simulink model "H8_6GDL_nolineal"  (R2022b)
settings: Solver=FixedStepAuto  StartTime=0.0  StopTime=5  FixedStep=1/7500  MaxStep=1e-3  RelTol=1e-3
InitFcn:
  | load("ems.mat");
  | load("hems.mat");
  | load('fuerzasY_LIM.mat')
  | load('matrices_linealizacion_6gdl.mat')
  | m = 200;
  | g = 9.81;
  | 
  | x_lev12 = 0.50086;
  | x_lev34 = 0.48414;
  | x_guid12 = 0.50503;
  | x_guid34 = 0.48831;
  | x_lim = 0.00778;
  | 
  | y_lev13 = 0.23523;
  | y_lev24 = 0.23827;
  | y_guid13 = 0.2372;
  | y_guid24 = 0.2402;
  | y_lim = 0.00154;
  | y_brk = 0.21552;
  | 
  | z_lev = 0.07138;
  | z_guid = 0.04113;
  | z_lim = 0.09146;
  | z_brk = 0.03941;
  | 
  | kp_lev = 50;
  | ki_lev = 400;
  | kp_guid = 6;
  | ki_guid = 46.5;
  | 
  | Imax_lev = 50;
  | Imin_lev = -50;
  | Imax_guid = 50;
  | Imin_guid = 0;
  | 
  | cg_nom=0.61448;
  | lev_nom=0.01965;
  | cg_suelo=0.61733;
  | cg_techo=0.60483;
  | 
  | I = [43.082 0 0; 0 26.887 -0; 0 0 29.297];
  | 
  | fs_current = 20000;
  | fl_current = 10000;
  | var_current = 0.052125100064495;
  | offset_current = 0.001065378087271;
  | 
  | fs_airgap = 20000;
  | fl_airgap = 7500;
  | var_airgap = 1.112140361208638e-08;
  | offset_airgap = 0;
  | airgap_min = 80/1000;
  | airgap_max = 115/1000;
  | 
  | current_filter_order = 20;
  | 
  | airgap_filter_order = 20;
  | N=16;
values from neighbouring files (symbols this model uses):
  A6 = [0 0 0 0 0 0 0 0 0 0 0 0 ... (100 elements, 10x10)]    [matrices_linealizacion_6gdl.mat]    (also in matrices_linealizacion_6gdl2.mat)
  B6 = [0 0 0 0 0 0 -0.0459993641186 -0.0505798680894 0.151580453785 0 0 0 ... (80 elements, 10x8)]    [matrices_linealizacion_6gdl.mat]    (also in matrices_linealizacion_6gdl2.mat)
  C6 = [1 0 0 0 0 0 0 0 0 0 0 1 ... (100 elements, 10x10)]    [matrices_linealizacion_6gdl.mat]    (also in matrices_linealizacion_6gdl2.mat)
  current = [0 10 20 30 40 50 60 70 80 90 100]    [fuerzasY_LIM.mat]
  D6 = [0 0 0 0 0 0 0 0 0 0 0 0 ... (80 elements, 10x8)]    [matrices_linealizacion_6gdl.mat]    (also in matrices_linealizacion_6gdl2.mat)
  FuerzaRail_Y = [0 0 0 0 0 0 0 0.015951701 0.168531476 0.364402347 0.577209778 0.832001165 ... (77 elements, 7x11)]    [fuerzasY_LIM.mat]
  hems =     [hems.mat]
  Ka = [0 0 0 0 4539.83149439 -4539.83149439 4539.83149439 -4539.83149439 -5130.48383819 -5130.48383819 -5130.48383819 -5130.48383819 ... (120 elements, 8x15)]    [Ka_reajustada.mat]    (also in matrices_linealizacion_6gdl.mat = [0 0 0 0 6002.75566687 -6002.75566687 6002.75566687 -6002.75; matrices_linealizacion_6gdl2.mat = [0 0 0 0 1200.55113337 -1200.55113337 1200.55113337 -1200.55)
  Y = [0 1 2 3 4 5 6]    [fuerzasY_LIM.mat]
undefined symbols (not defined in the file or in its folder): DiscIntNeverNeededParam, ems, magnitude
libraries: slpidlib x16, simulink x5
(part 2 of 2)

== system H8_6GDL_nolineal/EMS/RL ==
  target voltage : Inport
  airgap : Inport  Port=2
  temperature : Inport  Port=3
  2-D Lookup Table : Lookup_n-D  BreakpointsForDimension1=ems.Airgap  BreakpointsForDimension2=ems.Flux_Current(2:55)  Table=ems.Inductance  InternalRulePriority=Speed  RndMeth=Simplest
      settings: InputPortMap=u0,u1
  Abs : Abs  SaturateOnIntegerOverflow=off
  Add : Sum  Inputs=+-
  Delay{,1..3} (4 alike) : Delay  DelayLength=1
  Divide : Product  Inputs=*/
  Divide1 : Product  Inputs=*/
  Divide2 : Product  Inputs=*/
  Integrator1 : Integrator
  Subsystem : Subsystem
  to mm : Gain  Gain=1000
  current : Outport
  wires:
  airgap/1 -> to mm/1
  Divide/1 -> Integrator1/1
  Add/1 -> Divide/1
  Integrator1/1 -> Abs/1, current/1, Delay3/1, Add/2  "current applied"
  2-D Lookup Table/1 -> Divide2/1  "L"
  target voltage/1 -> Divide1/1
  temperature/1 -> Delay2/1
  Divide1/1 -> Add/1
  Subsystem/1(R) -> Divide2/2, Divide1/2  "R"
  Delay3/1 -> Subsystem/1(Current)
  Delay2/1 -> Subsystem/2(Temperature)
  Divide2/1 -> Divide/2
  Delay1/1 -> 2-D Lookup Table/2
  Delay/1 -> 2-D Lookup Table/1
  Abs/1 -> Delay1/1
  to mm/1 -> Delay/1

== system H8_6GDL_nolineal/EMS/RL1 ==
  target voltage : Inport
  airgap : Inport  Port=2
  temperature : Inport  Port=3
  2-D Lookup Table : Lookup_n-D  BreakpointsForDimension1=ems.Airgap  BreakpointsForDimension2=ems.Flux_Current(2:55)  Table=ems.Inductance  InternalRulePriority=Speed  RndMeth=Simplest
      settings: InputPortMap=u0,u1
  Abs : Abs  SaturateOnIntegerOverflow=off
  Add : Sum  Inputs=+-
  Delay{,1..3} (4 alike) : Delay  DelayLength=1
  Divide : Product  Inputs=*/
  Divide1 : Product  Inputs=*/
  Divide2 : Product  Inputs=*/
  Integrator1 : Integrator
  Subsystem : Subsystem
  to mm : Gain  Gain=1000
  current : Outport
  wires:
  airgap/1 -> to mm/1
  Divide/1 -> Integrator1/1
  Add/1 -> Divide/1
  Integrator1/1 -> Abs/1, current/1, Delay3/1, Add/2  "current applied"
  2-D Lookup Table/1 -> Divide2/1  "L"
  target voltage/1 -> Divide1/1
  temperature/1 -> Delay2/1
  Divide1/1 -> Add/1
  Subsystem/1(R) -> Divide2/2, Divide1/2  "R"
  Delay3/1 -> Subsystem/1(Current)
  Delay2/1 -> Subsystem/2(Temperature)
  Divide2/1 -> Divide/2
  Delay1/1 -> 2-D Lookup Table/2
  Delay/1 -> 2-D Lookup Table/1
  Abs/1 -> Delay1/1
  to mm/1 -> Delay/1

== system H8_6GDL_nolineal/EMS/RL2 ==
  target voltage : Inport
  airgap : Inport  Port=2
  temperature : Inport  Port=3
  2-D Lookup Table : Lookup_n-D  BreakpointsForDimension1=ems.Airgap  BreakpointsForDimension2=ems.Flux_Current(2:55)  Table=ems.Inductance  InternalRulePriority=Speed  RndMeth=Simplest
      settings: InputPortMap=u0,u1
  Abs : Abs  SaturateOnIntegerOverflow=off
  Add : Sum  Inputs=+-
  Delay{,1..3} (4 alike) : Delay  DelayLength=1
  Divide : Product  Inputs=*/
  Divide1 : Product  Inputs=*/
  Divide2 : Product  Inputs=*/
  Integrator1 : Integrator
  Subsystem : Subsystem
  to mm : Gain  Gain=1000
  current : Outport
  wires:
  airgap/1 -> to mm/1
  Divide/1 -> Integrator1/1
  Add/1 -> Divide/1
  Integrator1/1 -> Abs/1, current/1, Delay3/1, Add/2  "current applied"
  2-D Lookup Table/1 -> Divide2/1  "L"
  target voltage/1 -> Divide1/1
  temperature/1 -> Delay2/1
  Divide1/1 -> Add/1
  Subsystem/1(R) -> Divide2/2, Divide1/2  "R"
  Delay3/1 -> Subsystem/1(Current)
  Delay2/1 -> Subsystem/2(Temperature)
  Divide2/1 -> Divide/2
  Delay1/1 -> 2-D Lookup Table/2
  Delay/1 -> 2-D Lookup Table/1
  Abs/1 -> Delay1/1
  to mm/1 -> Delay/1

== system H8_6GDL_nolineal/EMS/RL3 ==
  target voltage : Inport
  airgap : Inport  Port=2
  temperature : Inport  Port=3
  2-D Lookup Table : Lookup_n-D  BreakpointsForDimension1=ems.Airgap  BreakpointsForDimension2=ems.Flux_Current(2:55)  Table=ems.Inductance  InternalRulePriority=Speed  RndMeth=Simplest
      settings: InputPortMap=u0,u1
  Abs : Abs  SaturateOnIntegerOverflow=off
  Add : Sum  Inputs=+-
  Delay{,1..3} (4 alike) : Delay  DelayLength=1
  Divide : Product  Inputs=*/
  Divide1 : Product  Inputs=*/
  Divide2 : Product  Inputs=*/
  Integrator1 : Integrator
  Subsystem : Subsystem
  to mm : Gain  Gain=1000
  current : Outport
  wires:
  airgap/1 -> to mm/1
  Divide/1 -> Integrator1/1
  Add/1 -> Divide/1
  Integrator1/1 -> Abs/1, current/1, Delay3/1, Add/2  "current applied"
  2-D Lookup Table/1 -> Divide2/1  "L"
  target voltage/1 -> Divide1/1
  temperature/1 -> Delay2/1
  Divide1/1 -> Add/1
  Subsystem/1(R) -> Divide2/2, Divide1/2  "R"
  Delay3/1 -> Subsystem/1(Current)
  Delay2/1 -> Subsystem/2(Temperature)
  Divide2/1 -> Divide/2
  Delay1/1 -> 2-D Lookup Table/2
  Delay/1 -> 2-D Lookup Table/1
  Abs/1 -> Delay1/1
  to mm/1 -> Delay/1

== system H8_6GDL_nolineal/EMS/Subsystem1 ==
  current5 : Inport
  Constant : Constant  Value=0
  Constant2 : Constant  Value=50
  Switch : Switch  Criteria=u2 > Threshold  SaturateOnIntegerOverflow=off  InputSameDT=off
  Switch1 : Switch  Criteria=u2 > Threshold  Threshold=50  SaturateOnIntegerOverflow=off  InputSameDT=off
  Out1 : Outport
  wires:
  current5/1 -> Switch/1, Switch/2
  Switch1/1 -> Out1/1
  Switch/1 -> Switch1/3, Switch1/2
  Constant/1 -> Switch/3
  Constant2/1 -> Switch1/1

== system H8_6GDL_nolineal/HEMS1/RL ==
  target voltage : Inport
  airgap : Inport  Port=2
  temperature : Inport  Port=3
  2-D Lookup Table : Lookup_n-D  BreakpointsForDimension1=hems.Airgap  BreakpointsForDimension2=hems.Current(2:110)  Table=hems.Inductance  InternalRulePriority=Speed  RndMeth=Simplest
      settings: InputPortMap=u0,u1
  Add : Sum  Inputs=+-
  Delay{1..4} (4 alike) : Delay  DelayLength=1
  Divide : Product  Inputs=*/
  Divide1 : Product  Inputs=*/
  Divide2 : Product  Inputs=*/
  Integrator1 : Integrator
  Rate Transition : RateTransition  Commented=through
  Saturation5 : Saturate  UpperLimit=0.0225  LowerLimit=0.01
  Subsystem : Subsystem
  to mm : Gain  Gain=1000
  current : Outport
  wires:
  airgap/1 -> Saturation5/1
  Divide/1 -> Integrator1/1
  Add/1 -> Divide/1
  Integrator1/1 -> Delay1/1, current/1, Delay3/1, Add/2  "current applied"
  2-D Lookup Table/1 -> Divide2/1  "L"
  temperature/1 -> Delay2/1
  Divide1/1 -> Add/1
  Subsystem/1(R) -> Divide2/2, Divide1/2  "R"
  Delay3/1 -> Subsystem/1(Current)
  Delay2/1 -> Subsystem/2(Temperature)
  Divide2/1 -> Divide/2
  Delay1/1 -> 2-D Lookup Table/2
  Rate Transition/1 -> 2-D Lookup Table/1
  Saturation5/1 -> to mm/1
  to mm/1 -> Delay4/1
  Delay4/1 -> Rate Transition/1
  target voltage/1 -> Divide1/1

== system H8_6GDL_nolineal/HEMS1/RL1 ==
  target current : Inport
  airgap : Inport  Port=2
  temperature : Inport  Port=3
  2-D Lookup Table : Lookup_n-D  BreakpointsForDimension1=hems.Airgap  BreakpointsForDimension2=hems.Current(2:110)  Table=hems.Inductance  InternalRulePriority=Speed  RndMeth=Simplest
      settings: InputPortMap=u0,u1
  Add : Sum  Inputs=+-
  Delay{1..4} (4 alike) : Delay  DelayLength=1
  Divide : Product  Inputs=*/
  Divide1 : Product  Inputs=*/
  Divide2 : Product  Inputs=*/
  Integrator1 : Integrator
  Rate Transition : RateTransition  Commented=through
  Saturation1 : Saturate  UpperLimit=0.0225  LowerLimit=0.01
  Subsystem : Subsystem
  to mm : Gain  Gain=1000
  current : Outport
  wires:
  airgap/1 -> Saturation1/1
  Divide/1 -> Integrator1/1
  Add/1 -> Divide/1
  Integrator1/1 -> Delay1/1, current/1, Delay3/1, Add/2  "current applied"
  2-D Lookup Table/1 -> Divide2/1  "L"
  target current/1 -> Divide1/1
  temperature/1 -> Delay2/1
  Divide1/1 -> Add/1
  Subsystem/1(R) -> Divide2/2, Divide1/2  "R"
  Delay3/1 -> Subsystem/1(Current)
  Delay2/1 -> Subsystem/2(Temperature)
  Divide2/1 -> Divide/2
  Delay1/1 -> 2-D Lookup Table/2
  Rate Transition/1 -> 2-D Lookup Table/1
  Saturation1/1 -> to mm/1
  to mm/1 -> Delay4/1
  Delay4/1 -> Rate Transition/1

== system H8_6GDL_nolineal/HEMS1/RL2 ==
  target current : Inport
  airgap : Inport  Port=2
  temperature : Inport  Port=3
  2-D Lookup Table : Lookup_n-D  BreakpointsForDimension1=hems.Airgap  BreakpointsForDimension2=hems.Current(2:110)  Table=hems.Inductance  InternalRulePriority=Speed  RndMeth=Simplest
      settings: InputPortMap=u0,u1
  Add : Sum  Inputs=+-
  Delay{1..4} (4 alike) : Delay  DelayLength=1
  Divide : Product  Inputs=*/
  Divide1 : Product  Inputs=*/
  Divide2 : Product  Inputs=*/
  Integrator1 : Integrator
  Rate Transition : RateTransition  Commented=through
  Saturation5 : Saturate  UpperLimit=0.0225  LowerLimit=0.01
  Subsystem : Subsystem
  to mm : Gain  Gain=1000
  current : Outport
  wires:
  airgap/1 -> Saturation5/1
  Divide/1 -> Integrator1/1
  Add/1 -> Divide/1
  Integrator1/1 -> Delay1/1, current/1, Delay3/1, Add/2  "current applied"
  2-D Lookup Table/1 -> Divide2/1  "L"
  target current/1 -> Divide1/1
  temperature/1 -> Delay2/1
  Divide1/1 -> Add/1
  Subsystem/1(R) -> Divide2/2, Divide1/2  "R"
  Delay3/1 -> Subsystem/1(Current)
  Delay2/1 -> Subsystem/2(Temperature)
  Divide2/1 -> Divide/2
  Delay1/1 -> 2-D Lookup Table/2
  Rate Transition/1 -> 2-D Lookup Table/1
  Saturation5/1 -> to mm/1
  to mm/1 -> Delay4/1
  Delay4/1 -> Rate Transition/1

== system H8_6GDL_nolineal/HEMS1/RL3 ==
  target current : Inport
  airgap : Inport  Port=2
  temperature : Inport  Port=3
  2-D Lookup Table : Lookup_n-D  BreakpointsForDimension1=hems.Airgap  BreakpointsForDimension2=hems.Current(2:110)  Table=hems.Inductance  InternalRulePriority=Speed  RndMeth=Simplest
      settings: InputPortMap=u0,u1
  Add : Sum  Inputs=+-
  Delay{1..4} (4 alike) : Delay  DelayLength=1
  Divide : Product  Inputs=*/
  Divide1 : Product  Inputs=*/
  Divide2 : Product  Inputs=*/
  Integrator1 : Integrator
  Rate Transition : RateTransition  Commented=through
  Saturation5 : Saturate  UpperLimit=0.0225  LowerLimit=0.01
  Subsystem : Subsystem
  to mm : Gain  Gain=1000
  current : Outport
  wires:
  airgap/1 -> Saturation5/1
  Divide/1 -> Integrator1/1
  Add/1 -> Divide/1
  Integrator1/1 -> Delay1/1, current/1, Delay3/1, Add/2  "current applied"
  2-D Lookup Table/1 -> Divide2/1  "L"
  target current/1 -> Divide1/1
  temperature/1 -> Delay2/1
  Divide1/1 -> Add/1
  Subsystem/1(R) -> Divide2/2, Divide1/2  "R"
  Delay3/1 -> Subsystem/1(Current)
  Delay2/1 -> Subsystem/2(Temperature)
  Divide2/1 -> Divide/2
  Delay1/1 -> 2-D Lookup Table/2
  Rate Transition/1 -> 2-D Lookup Table/1
  Saturation5/1 -> to mm/1
  to mm/1 -> Delay4/1
  Delay4/1 -> Rate Transition/1

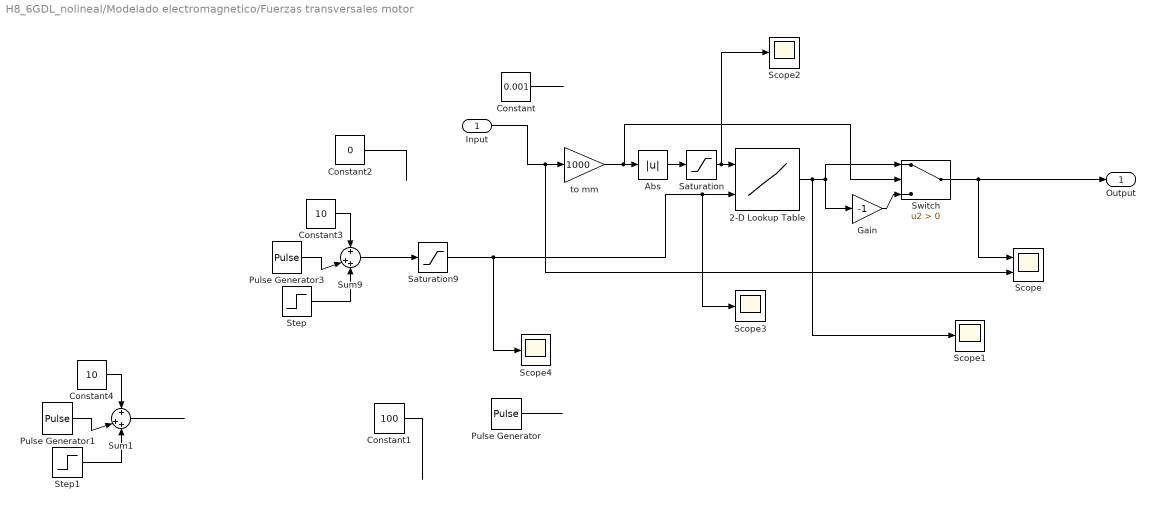
== system H8_6GDL_nolineal/Modelado electromagnetico/Fuerzas transversales motor ==
  Input : Inport
  2-D Lookup Table : Lookup_n-D  BreakpointsForDimension1=Y  BreakpointsForDimension2=current  Table=FuerzaRail_Y  InternalRulePriority=Speed  RndMeth=Simplest
      settings: InputPortMap=u0,u1
  Abs : Abs  SaturateOnIntegerOverflow=off
  Constant : Constant  Value=0.001
  Constant1 : Constant  Value=100
  Constant2 : Constant  Value=0
  Constant3 : Constant  Value=10
  Constant4 : Constant  Value=10
  Gain : Gain  Gain=-1
  Pulse Generator : DiscretePulseGenerator  PulseType=Time based  Amplitude=100  PulseWidth=75  PhaseDelay=3
  Pulse Generator1 : DiscretePulseGenerator  PulseType=Time based  Amplitude=100  PulseWidth=95  PhaseDelay=4.2
  Pulse Generator3 : DiscretePulseGenerator  PulseType=Time based  Amplitude=100  PulseWidth=95  PhaseDelay=1
  Saturation : Saturate  UpperLimit=6  LowerLimit=0
  Saturation9 : Saturate  UpperLimit=100  LowerLimit=0
  Scope : Scope  NumInputPorts=2
  Scope{1..4} (4 alike) : Scope
  Step : Step  Time=5  After=-100  SampleTime=0
  Step1 : Step  Time=8.2  After=-100  SampleTime=0
  Sum1 : Sum  Inputs=+|++
  Sum9 : Sum  Inputs=+|++
  Switch : Switch  Criteria=u2 > Threshold  SaturateOnIntegerOverflow=off  InputSameDT=off
  to mm : Gain  Gain=1000
  Output : Outport
  wires:
  Constant/1 -> ?
  Input/1 -> to mm/1, Scope/2
  Gain/1 -> Switch/3
  Abs/1 -> Saturation/1
  to mm/1 -> Switch/2, Abs/1
  2-D Lookup Table/1 -> Scope1/1, Gain/1, Switch/1
  Saturation9/1 -> Scope4/1, Scope3/1, 2-D Lookup Table/2
  Switch/1 -> Output/1, Scope/1
  Saturation/1 -> Scope2/1, 2-D Lookup Table/1
  Pulse Generator/1 -> ?
  Constant1/1 -> ?
  Constant2/1 -> ?
  Sum9/1 -> Saturation9/1
  Pulse Generator3/1 -> Sum9/2
  Constant3/1 -> Sum9/1
  Step/1 -> Sum9/3
  Constant4/1 -> Sum1/1
  Step1/1 -> Sum1/3
  Pulse Generator1/1 -> Sum1/2
  Sum1/1 -> ?

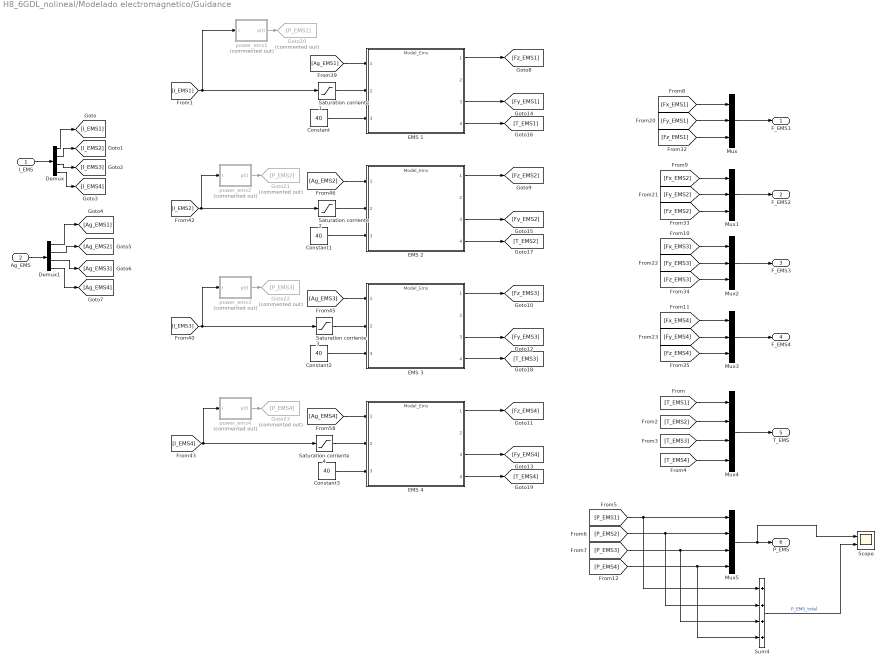
== system H8_6GDL_nolineal/Modelado electromagnetico/Guidance ==
  I_EMS : Inport
  Ag_EMS : Inport  Port=2
  Constant{,1..3} (4 alike) : Constant  Value=40
  Demux : Demux
  Demux1 : Demux
  EMS {1..4} (4 alike) : ModelReference  ModelNameDialog=Model_Ems.slx  SimulationMode=Normal  ModelReferenceVersion=1.24
  Goto20 : Goto  Commented=on  GotoTag=P_EMS1
  Goto21 : Goto  Commented=on  GotoTag=P_EMS2
  Goto22 : Goto  Commented=on  GotoTag=P_EMS3
  Goto23 : Goto  Commented=on  GotoTag=P_EMS4
  Mux{,1..3} (4 alike) : Mux  Inputs=3
  Mux4 : Mux
  Mux5 : Mux
  Saturation corriente {1..4} (4 alike) : Saturate  UpperLimit=Imax_guid  LowerLimit=Imin_guid
  Scope : Scope  NumInputPorts=2
  Sum4 : Sum  Inputs=++++
  power_ems1 : Subsystem  Commented=on
  power_ems2 : Subsystem  Commented=on
  power_ems3 : Subsystem  Commented=on
  power_ems4 : Subsystem  Commented=on
  F_EMS1 : Outport
  F_EMS2 : Outport  Port=2
  F_EMS3 : Outport  Port=3
  F_EMS4 : Outport  Port=4
  T_EMS : Outport  Port=5
  P_EMS : Outport  Port=6
  wires:
  [Fz_EMS4] -> Mux3/3
  Demux1/4 -> [Ag_EMS4]
  [Fy_EMS1] -> Mux/2
  I_EMS/1 -> Demux/1
  Mux1/1 -> F_EMS2/1
  Demux/2 -> [I_EMS2]
  [Fy_EMS3] -> Mux2/2
  Mux3/1 -> F_EMS4/1
  [Fy_EMS4] -> Mux3/2
  [Fz_EMS1] -> Mux/3
  Mux/1 -> F_EMS1/1
  Mux2/1 -> F_EMS3/1
  [Fx_EMS3] -> Mux2/1
  Demux1/3 -> [Ag_EMS3]
  Ag_EMS/1 -> Demux1/1
  [Fz_EMS3] -> Mux2/3
  Demux/1 -> [I_EMS1]
  [Fz_EMS2] -> Mux1/3
  [Fx_EMS1] -> Mux/1
  Demux1/1 -> [Ag_EMS1]
  Demux/4 -> [I_EMS4]
  [Fx_EMS2] -> Mux1/1
  [Fy_EMS2] -> Mux1/2
  [Fx_EMS4] -> Mux3/1
  Demux/3 -> [I_EMS3]
  Demux1/2 -> [Ag_EMS2]
  EMS 1/3 -> [Fy_EMS1]
  [Ag_EMS4] -> EMS 4/1
  EMS 4/3 -> [Fy_EMS4]
  EMS 4/1 -> [Fz_EMS4]
  EMS 2/1 -> [Fz_EMS2]
  EMS 3/1 -> [Fz_EMS3]
  [Ag_EMS3] -> EMS 3/1
  Constant1/1 -> EMS 2/3
  Constant3/1 -> EMS 4/3
  Constant2/1 -> EMS 3/3
  Constant/1 -> EMS 1/3
  EMS 1/1 -> [Fz_EMS1]
  [Ag_EMS2] -> EMS 2/1
  EMS 3/3 -> [Fy_EMS3]
  EMS 2/3 -> [Fy_EMS2]
  [Ag_EMS1] -> EMS 1/1
  Mux4/1 -> T_EMS/1
  EMS 1/4 -> [T_EMS1]
  EMS 2/4 -> [T_EMS2]
  EMS 3/4 -> [T_EMS3]
  EMS 4/4 -> [T_EMS4]
  [T_EMS1] -> Mux4/1
  [T_EMS2] -> Mux4/2
  [T_EMS3] -> Mux4/3
  [T_EMS4] -> Mux4/4
  Saturation corriente 1/1 -> EMS 1/2
  Saturation corriente 2/1 -> EMS 2/2
  Saturation corriente 3/1 -> EMS 3/2
  Saturation corriente 4/1 -> EMS 4/2
  power_ems1/1(p(t)) -> Goto20/1
  power_ems2/1(p(t)) -> Goto21/1
  power_ems3/1(p(t)) -> Goto22/1
  power_ems4/1(p(t)) -> Goto23/1
  [P_EMS4] -> Sum4/4, Mux5/4
  [P_EMS1] -> Mux5/1, Sum4/1
  Sum4/1 -> Scope/2  "P_EMS_total"
  [P_EMS2] -> Mux5/2, Sum4/2
  Mux5/1 -> Scope/1, P_EMS/1
  [P_EMS3] -> Sum4/3, Mux5/3
  [I_EMS4] -> Saturation corriente 4/1, power_ems4/1(I)
  [I_EMS3] -> Saturation corriente 3/1, power_ems3/1(I)
  [I_EMS2] -> Saturation corriente 2/1, power_ems2/1(I)
  [I_EMS1] -> Saturation corriente 1/1, power_ems1/1(I)

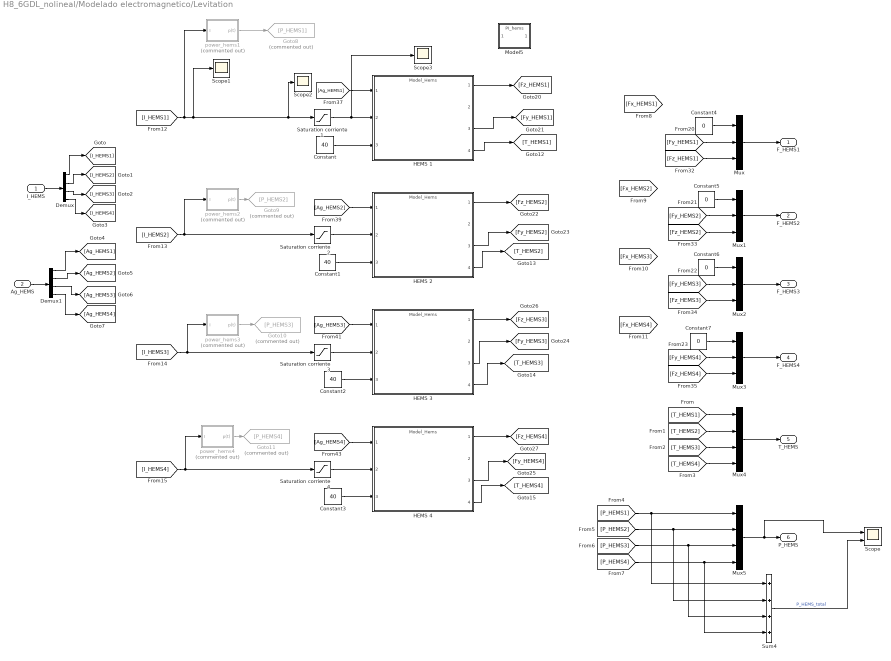
== system H8_6GDL_nolineal/Modelado electromagnetico/Levitation ==
  I_HEMS : Inport
  Ag_HEMS : Inport  Port=2
  Constant{,1..3} (4 alike) : Constant  Value=40
  Constant{4..7} (4 alike) : Constant  Value=0
  Demux : Demux
  Demux1 : Demux
  Goto10 : Goto  Commented=on  GotoTag=P_HEMS3
  Goto11 : Goto  Commented=on  GotoTag=P_HEMS4
  Goto8 : Goto  Commented=on  GotoTag=P_HEMS1
  Goto9 : Goto  Commented=on  GotoTag=P_HEMS2
  HEMS {1..4} (4 alike) : ModelReference  ModelNameDialog=Model_Hems.slx  SimulationMode=Normal  ModelReferenceVersion=1.27
  Model5 : ModelReference  ModelNameDialog=PI_hems.slx  SimulationMode=Normal  ModelReferenceVersion=1.6
  Mux{,1..3} (4 alike) : Mux  Inputs=3
  Mux4 : Mux
  Mux5 : Mux
  Saturation corriente {1..4} (4 alike) : Saturate  UpperLimit=Imax_lev  LowerLimit=Imin_lev
  Scope : Scope  NumInputPorts=2
  Scope1 : Scope
  Scope2 : Scope
  Scope3 : Scope
  Sum4 : Sum  Inputs=++++
  power_hems1 : Subsystem  Commented=on
  power_hems2 : Subsystem  Commented=on
  power_hems3 : Subsystem  Commented=on
  power_hems4 : Subsystem  Commented=on
  F_HEMS1 : Outport
  F_HEMS2 : Outport  Port=2
  F_HEMS3 : Outport  Port=3
  F_HEMS4 : Outport  Port=4
  T_HEMS : Outport  Port=5
  P_HEMS : Outport  Port=6
  wires:
  I_HEMS/1 -> Demux/1
  Mux/1 -> F_HEMS1/1
  Mux1/1 -> F_HEMS2/1
  Mux2/1 -> F_HEMS3/1
  Mux3/1 -> F_HEMS4/1
  Demux/1 -> [I_HEMS1]
  Demux/2 -> [I_HEMS2]
  Demux/3 -> [I_HEMS3]
  Demux/4 -> [I_HEMS4]
  Demux1/2 -> [Ag_HEMS2]
  Demux1/3 -> [Ag_HEMS3]
  Ag_HEMS/1 -> Demux1/1
  Demux1/4 -> [Ag_HEMS4]
  Demux1/1 -> [Ag_HEMS1]
  Constant4/1 -> Mux/1
  Constant5/1 -> Mux1/1
  Constant6/1 -> Mux2/1
  Constant7/1 -> Mux3/1
  [Fy_HEMS1] -> Mux/2
  [Fy_HEMS2] -> Mux1/2
  [Fy_HEMS3] -> Mux2/2
  [Fy_HEMS4] -> Mux3/2
  [Fz_HEMS1] -> Mux/3
  [Fz_HEMS2] -> Mux1/3
  [Fz_HEMS3] -> Mux2/3
  [Fz_HEMS4] -> Mux3/3
  [Ag_HEMS1] -> HEMS 1/1
  HEMS 1/1 -> [Fz_HEMS1]
  HEMS 1/3 -> [Fy_HEMS1]
  HEMS 2/3 -> [Fy_HEMS2]
  HEMS 2/1 -> [Fz_HEMS2]
  [Ag_HEMS2] -> HEMS 2/1
  HEMS 3/3 -> [Fy_HEMS3]
  HEMS 3/1 -> [Fz_HEMS3]
  [Ag_HEMS3] -> HEMS 3/1
  HEMS 4/3 -> [Fy_HEMS4]
  HEMS 4/1 -> [Fz_HEMS4]
  [Ag_HEMS4] -> HEMS 4/1
  Constant1/1 -> HEMS 2/3
  Constant2/1 -> HEMS 3/3
  Constant3/1 -> HEMS 4/3
  HEMS 1/4 -> [T_HEMS1]
  Constant/1 -> HEMS 1/3
  HEMS 2/4 -> [T_HEMS2]
  HEMS 3/4 -> [T_HEMS3]
  HEMS 4/4 -> [T_HEMS4]
  Mux4/1 -> T_HEMS/1
  [T_HEMS1] -> Mux4/1
  [T_HEMS4] -> Mux4/4
  [T_HEMS3] -> Mux4/3
  [T_HEMS2] -> Mux4/2
  Saturation corriente 1/1 -> Scope3/1, HEMS 1/2
  Saturation corriente 2/1 -> HEMS 2/2
  Saturation corriente 3/1 -> HEMS 3/2
  Saturation corriente 4/1 -> HEMS 4/2
  power_hems1/1(p(t)) -> Goto8/1
  [P_HEMS4] -> Sum4/4, Mux5/4
  [P_HEMS2] -> Mux5/2, Sum4/2
  [P_HEMS3] -> Sum4/3, Mux5/3
  Mux5/1 -> Scope/1, P_HEMS/1
  [P_HEMS1] -> Mux5/1, Sum4/1
  Sum4/1 -> Scope/2  "P_HEMS_total"
  power_hems2/1(p(t)) -> Goto9/1
  power_hems3/1(p(t)) -> Goto10/1
  power_hems4/1(p(t)) -> Goto11/1
  [I_HEMS4] -> Saturation corriente 4/1, power_hems4/1(I)
  [I_HEMS2] -> Saturation corriente 2/1, power_hems2/1(I)
  [I_HEMS1] -> power_hems1/1(I), Scope2/1, Saturation corriente 1/1, Scope1/1
  [I_HEMS3] -> Saturation corriente 3/1, power_hems3/1(I)

== system H8_6GDL_nolineal/Subsystem/Discr_Ampl ==
  señal : Inport
  Constant : Constant  Value=N
  Constant1 : Constant  Value=Max
  Constant2 : Constant  Value=Min
  MATLAB Function1 : MATLAB Function  TreatAsAtomicUnit=on
  señal_discretizada : Outport
  wires:
  MATLAB Function1/1(senal_discretizada) -> señal_discretizada/1
  señal/1 -> MATLAB Function1/1(senal)
  Constant1/1 -> MATLAB Function1/3(Max)
  Constant/1 -> MATLAB Function1/2(N)
  Constant2/1 -> MATLAB Function1/4(Min)

== system H8_6GDL_nolineal/Subsystem/Discr_Ampl1 ==
  señal : Inport
  Constant : Constant  Value=N
  Constant1 : Constant  Value=Max
  Constant2 : Constant  Value=Min
  MATLAB Function1 : MATLAB Function  TreatAsAtomicUnit=on
  señal_discretizada : Outport
  wires:
  MATLAB Function1/1(senal_discretizada) -> señal_discretizada/1
  señal/1 -> MATLAB Function1/1(senal)
  Constant1/1 -> MATLAB Function1/3(Max)
  Constant/1 -> MATLAB Function1/2(N)
  Constant2/1 -> MATLAB Function1/4(Min)

== system H8_6GDL_nolineal/Subsystem/Discr_Ampl2 ==
  señal : Inport
  Constant : Constant  Value=N
  Constant1 : Constant  Value=Max
  Constant2 : Constant  Value=Min
  MATLAB Function1 : MATLAB Function  TreatAsAtomicUnit=on
  señal_discretizada : Outport
  wires:
  MATLAB Function1/1(senal_discretizada) -> señal_discretizada/1
  señal/1 -> MATLAB Function1/1(senal)
  Constant1/1 -> MATLAB Function1/3(Max)
  Constant/1 -> MATLAB Function1/2(N)
  Constant2/1 -> MATLAB Function1/4(Min)

== system H8_6GDL_nolineal/Subsystem/Discr_Ampl3 ==
  señal : Inport
  Constant : Constant  Value=N
  Constant1 : Constant  Value=Max
  Constant2 : Constant  Value=Min
  MATLAB Function1 : MATLAB Function  TreatAsAtomicUnit=on
  señal_discretizada : Outport
  wires:
  MATLAB Function1/1(senal_discretizada) -> señal_discretizada/1
  señal/1 -> MATLAB Function1/1(senal)
  Constant1/1 -> MATLAB Function1/3(Max)
  Constant/1 -> MATLAB Function1/2(N)
  Constant2/1 -> MATLAB Function1/4(Min)

== system H8_6GDL_nolineal/Subsystem/Discr_Ampl4 ==
  señal : Inport
  Constant : Constant  Value=N
  Constant1 : Constant  Value=Max
  Constant2 : Constant  Value=Min
  MATLAB Function1 : MATLAB Function  TreatAsAtomicUnit=on
  señal_discretizada : Outport
  wires:
  MATLAB Function1/1(senal_discretizada) -> señal_discretizada/1
  señal/1 -> MATLAB Function1/1(senal)
  Constant1/1 -> MATLAB Function1/3(Max)
  Constant/1 -> MATLAB Function1/2(N)
  Constant2/1 -> MATLAB Function1/4(Min)

== system H8_6GDL_nolineal/Subsystem/Discr_Ampl5 ==
  señal : Inport
  Constant : Constant  Value=N
  Constant1 : Constant  Value=Max
  Constant2 : Constant  Value=Min
  MATLAB Function1 : MATLAB Function  TreatAsAtomicUnit=on
  señal_discretizada : Outport
  wires:
  MATLAB Function1/1(senal_discretizada) -> señal_discretizada/1
  señal/1 -> MATLAB Function1/1(senal)
  Constant1/1 -> MATLAB Function1/3(Max)
  Constant/1 -> MATLAB Function1/2(N)
  Constant2/1 -> MATLAB Function1/4(Min)

== system H8_6GDL_nolineal/Subsystem/Discr_Ampl6 ==
  señal : Inport
  Constant : Constant  Value=N
  Constant1 : Constant  Value=Max
  Constant2 : Constant  Value=Min
  MATLAB Function1 : MATLAB Function  TreatAsAtomicUnit=on
  señal_discretizada : Outport
  wires:
  MATLAB Function1/1(senal_discretizada) -> señal_discretizada/1
  señal/1 -> MATLAB Function1/1(senal)
  Constant1/1 -> MATLAB Function1/3(Max)
  Constant/1 -> MATLAB Function1/2(N)
  Constant2/1 -> MATLAB Function1/4(Min)

== system H8_6GDL_nolineal/Subsystem/Discr_Ampl7 ==
  señal : Inport
  Constant : Constant  Value=N
  Constant1 : Constant  Value=Max
  Constant2 : Constant  Value=Min
  MATLAB Function1 : MATLAB Function  TreatAsAtomicUnit=on
  señal_discretizada : Outport
  wires:
  MATLAB Function1/1(senal_discretizada) -> señal_discretizada/1
  señal/1 -> MATLAB Function1/1(senal)
  Constant1/1 -> MATLAB Function1/3(Max)
  Constant/1 -> MATLAB Function1/2(N)
  Constant2/1 -> MATLAB Function1/4(Min)

== system H8_6GDL_nolineal/Subsystem/Moving Average Filter ==
  input : Inport
  Delay : Delay  DelayLength=M  SampleTime=fs
  Delay1 : Delay  DelayLength=1  SampleTime=fs
  Gain : Gain  Gain=1/M
  Sum : Sum  Inputs=|+-
  Sum1 : Sum  Inputs=|++
  output : Outport
  wires:
  input/1 -> Delay/1, Sum/1
  Delay/1 -> Sum/2
  Sum/1 -> Sum1/1
  Sum1/1 -> Delay1/1, Gain/1
  Delay1/1 -> Sum1/2
  Gain/1 -> output/1

== system H8_6GDL_nolineal/Subsystem/Moving Average Filter1 ==
  input : Inport
  Delay : Delay  DelayLength=M  SampleTime=fs
  Delay1 : Delay  DelayLength=1  SampleTime=fs
  Gain : Gain  Gain=1/M
  Sum : Sum  Inputs=|+-
  Sum1 : Sum  Inputs=|++
  output : Outport
  wires:
  input/1 -> Delay/1, Sum/1
  Delay/1 -> Sum/2
  Sum/1 -> Sum1/1
  Sum1/1 -> Delay1/1, Gain/1
  Delay1/1 -> Sum1/2
  Gain/1 -> output/1

== system H8_6GDL_nolineal/Subsystem/Moving Average Filter2 ==
  input : Inport
  Delay : Delay  DelayLength=M  SampleTime=fs
  Delay1 : Delay  DelayLength=1  SampleTime=fs
  Gain : Gain  Gain=1/M
  Sum : Sum  Inputs=|+-
  Sum1 : Sum  Inputs=|++
  output : Outport
  wires:
  input/1 -> Delay/1, Sum/1
  Delay/1 -> Sum/2
  Sum/1 -> Sum1/1
  Sum1/1 -> Delay1/1, Gain/1
  Delay1/1 -> Sum1/2
  Gain/1 -> output/1

== system H8_6GDL_nolineal/Subsystem/Moving Average Filter3 ==
  input : Inport
  Delay : Delay  DelayLength=M  SampleTime=fs
  Delay1 : Delay  DelayLength=1  SampleTime=fs
  Gain : Gain  Gain=1/M
  Sum : Sum  Inputs=|+-
  Sum1 : Sum  Inputs=|++
  output : Outport
  wires:
  input/1 -> Delay/1, Sum/1
  Delay/1 -> Sum/2
  Sum/1 -> Sum1/1
  Sum1/1 -> Delay1/1, Gain/1
  Delay1/1 -> Sum1/2
  Gain/1 -> output/1

== system H8_6GDL_nolineal/Subsystem/Moving Average Filter4 ==
  input : Inport
  Delay : Delay  DelayLength=M  SampleTime=fs
  Delay1 : Delay  DelayLength=1  SampleTime=fs
  Gain : Gain  Gain=1/M
  Sum : Sum  Inputs=|+-
  Sum1 : Sum  Inputs=|++
  output : Outport
  wires:
  input/1 -> Delay/1, Sum/1
  Delay/1 -> Sum/2
  Sum/1 -> Sum1/1
  Sum1/1 -> Delay1/1, Gain/1
  Delay1/1 -> Sum1/2
  Gain/1 -> output/1

== system H8_6GDL_nolineal/Subsystem/Moving Average Filter5 ==
  input : Inport
  Delay : Delay  DelayLength=M  SampleTime=fs
  Delay1 : Delay  DelayLength=1  SampleTime=fs
  Gain : Gain  Gain=1/M
  Sum : Sum  Inputs=|+-
  Sum1 : Sum  Inputs=|++
  output : Outport
  wires:
  input/1 -> Delay/1, Sum/1
  Delay/1 -> Sum/2
  Sum/1 -> Sum1/1
  Sum1/1 -> Delay1/1, Gain/1
  Delay1/1 -> Sum1/2
  Gain/1 -> output/1

== system H8_6GDL_nolineal/Subsystem/Moving Average Filter6 ==
  input : Inport
  Delay : Delay  DelayLength=M  SampleTime=fs
  Delay1 : Delay  DelayLength=1  SampleTime=fs
  Gain : Gain  Gain=1/M
  Sum : Sum  Inputs=|+-
  Sum1 : Sum  Inputs=|++
  output : Outport
  wires:
  input/1 -> Delay/1, Sum/1
  Delay/1 -> Sum/2
  Sum/1 -> Sum1/1
  Sum1/1 -> Delay1/1, Gain/1
  Delay1/1 -> Sum1/2
  Gain/1 -> output/1

== system H8_6GDL_nolineal/Subsystem/Moving Average Filter7 ==
  input : Inport
  Delay : Delay  DelayLength=M  SampleTime=fs
  Delay1 : Delay  DelayLength=1  SampleTime=fs
  Gain : Gain  Gain=1/M
  Sum : Sum  Inputs=|+-
  Sum1 : Sum  Inputs=|++
  output : Outport
  wires:
  input/1 -> Delay/1, Sum/1
  Delay/1 -> Sum/2
  Sum/1 -> Sum1/1
  Sum1/1 -> Delay1/1, Gain/1
  Delay1/1 -> Sum1/2
  Gain/1 -> output/1

== system H8_6GDL_nolineal/Subsystem/Ruido ==
  Señal : Inport
  Random Number : RandomNumber  Commented=on  Mean=M  Variance=V  Seed=3  SampleTime=T
  Sum : Sum  Inputs=|++
  Señal_ruido : Outport
  wires:
  Random Number/1 -> Sum/2
  Señal/1 -> Sum/1
  Sum/1 -> Señal_ruido/1

== system H8_6GDL_nolineal/Subsystem/Ruido1 ==
  Señal : Inport
  Random Number : RandomNumber  Commented=on  Mean=M  Variance=V  Seed=3  SampleTime=T
  Sum : Sum  Inputs=|++
  Señal_ruido : Outport
  wires:
  Random Number/1 -> Sum/2
  Señal/1 -> Sum/1
  Sum/1 -> Señal_ruido/1

== system H8_6GDL_nolineal/Subsystem/Ruido2 ==
  Señal : Inport
  Random Number : RandomNumber  Commented=on  Mean=M  Variance=V  Seed=3  SampleTime=T
  Sum : Sum  Inputs=|++
  Señal_ruido : Outport
  wires:
  Random Number/1 -> Sum/2
  Señal/1 -> Sum/1
  Sum/1 -> Señal_ruido/1

== system H8_6GDL_nolineal/Subsystem/Ruido3 ==
  Señal : Inport
  Random Number : RandomNumber  Commented=on  Mean=M  Variance=V  Seed=3  SampleTime=T
  Sum : Sum  Inputs=|++
  Señal_ruido : Outport
  wires:
  Random Number/1 -> Sum/2
  Señal/1 -> Sum/1
  Sum/1 -> Señal_ruido/1

== system H8_6GDL_nolineal/Subsystem/Ruido4 ==
  Señal : Inport
  Random Number : RandomNumber  Commented=on  Mean=M  Variance=V  Seed=3  SampleTime=T
  Sum : Sum  Inputs=|++
  Señal_ruido : Outport
  wires:
  Random Number/1 -> Sum/2
  Señal/1 -> Sum/1
  Sum/1 -> Señal_ruido/1

== system H8_6GDL_nolineal/Subsystem/Ruido5 ==
  Señal : Inport
  Random Number : RandomNumber  Commented=on  Mean=M  Variance=V  Seed=3  SampleTime=T
  Sum : Sum  Inputs=|++
  Señal_ruido : Outport
  wires:
  Random Number/1 -> Sum/2
  Señal/1 -> Sum/1
  Sum/1 -> Señal_ruido/1

== system H8_6GDL_nolineal/Subsystem/Ruido6 ==
  Señal : Inport
  Random Number : RandomNumber  Mean=M  Variance=V  Seed=3  SampleTime=T
  Sum : Sum  Inputs=|++
  Señal_ruido : Outport
  wires:
  Random Number/1 -> Sum/2
  Señal/1 -> Sum/1
  Sum/1 -> Señal_ruido/1

== system H8_6GDL_nolineal/Subsystem/Ruido7 ==
  Señal : Inport
  Random Number : RandomNumber  Mean=M  Variance=V  Seed=3  SampleTime=T
  Sum : Sum  Inputs=|++
  Señal_ruido : Outport
  wires:
  Random Number/1 -> Sum/2
  Señal/1 -> Sum/1
  Sum/1 -> Señal_ruido/1

== system H8_6GDL_nolineal/Subsystem/Ruido8 ==
  Señal : Inport
  Random Number : RandomNumber  Mean=M  Variance=V  Seed=3  SampleTime=T
  Sum : Sum  Inputs=|++
  Señal_ruido : Outport
  wires:
  Random Number/1 -> Sum/2
  Señal/1 -> Sum/1
  Sum/1 -> Señal_ruido/1

== system H8_6GDL_nolineal/Control/state space control/Moving Average Filter ==
  input : Inport
  Delay : Delay  DelayLength=M  SampleTime=fs
  Delay1 : Delay  DelayLength=1  SampleTime=fs
  Gain : Gain  Gain=1/M
  Sum : Sum  Inputs=|+-
  Sum1 : Sum  Inputs=|++
  output : Outport
  wires:
  input/1 -> Delay/1, Sum/1
  Delay/1 -> Sum/2
  Sum/1 -> Sum1/1
  Sum1/1 -> Delay1/1, Gain/1
  Delay1/1 -> Sum1/2
  Gain/1 -> output/1

== system H8_6GDL_nolineal/Control/state space control/Moving Average Filter1 ==
  input : Inport
  Delay : Delay  DelayLength=M  SampleTime=fs
  Delay1 : Delay  DelayLength=1  SampleTime=fs
  Gain : Gain  Gain=1/M
  Sum : Sum  Inputs=|+-
  Sum1 : Sum  Inputs=|++
  output : Outport
  wires:
  input/1 -> Delay/1, Sum/1
  Delay/1 -> Sum/2
  Sum/1 -> Sum1/1
  Sum1/1 -> Delay1/1, Gain/1
  Delay1/1 -> Sum1/2
  Gain/1 -> output/1

== system H8_6GDL_nolineal/Control/state space control/Moving Average Filter2 ==
  input : Inport
  Delay : Delay  DelayLength=M  SampleTime=fs
  Delay1 : Delay  DelayLength=1  SampleTime=fs
  Gain : Gain  Gain=1/M
  Sum : Sum  Inputs=|+-
  Sum1 : Sum  Inputs=|++
  output : Outport
  wires:
  input/1 -> Delay/1, Sum/1
  Delay/1 -> Sum/2
  Sum/1 -> Sum1/1
  Sum1/1 -> Delay1/1, Gain/1
  Delay1/1 -> Sum1/2
  Gain/1 -> output/1

== system H8_6GDL_nolineal/Control/state space control/Moving Average Filter3 ==
  input : Inport
  Delay : Delay  DelayLength=M  SampleTime=fs
  Delay1 : Delay  DelayLength=1  SampleTime=fs
  Gain : Gain  Gain=1/M
  Sum : Sum  Inputs=|+-
  Sum1 : Sum  Inputs=|++
  output : Outport
  wires:
  input/1 -> Delay/1, Sum/1
  Delay/1 -> Sum/2
  Sum/1 -> Sum1/1
  Sum1/1 -> Delay1/1, Gain/1
  Delay1/1 -> Sum1/2
  Gain/1 -> output/1

== system H8_6GDL_nolineal/Control/state space control/Moving Average Filter4 ==
  input : Inport
  Delay : Delay  DelayLength=M  SampleTime=fs
  Delay1 : Delay  DelayLength=1  SampleTime=fs
  Gain : Gain  Gain=1/M
  Sum : Sum  Inputs=|+-
  Sum1 : Sum  Inputs=|++
  output : Outport
  wires:
  input/1 -> Delay/1, Sum/1
  Delay/1 -> Sum/2
  Sum/1 -> Sum1/1
  Sum1/1 -> Delay1/1, Gain/1
  Delay1/1 -> Sum1/2
  Gain/1 -> output/1

== system H8_6GDL_nolineal/EMS/RL/Subsystem ==
  Current : Inport
  Temperature : Inport  Port=2
  Resistance : Constant  Value=ems.Resistance
  R : Outport
  wires:
  Resistance/1 -> R/1

== system H8_6GDL_nolineal/EMS/RL1/Subsystem ==
  Current : Inport
  Temperature : Inport  Port=2
  Resistance : Constant  Value=ems.Resistance
  R : Outport
  wires:
  Resistance/1 -> R/1

== system H8_6GDL_nolineal/EMS/RL2/Subsystem ==
  Current : Inport
  Temperature : Inport  Port=2
  Resistance : Constant  Value=ems.Resistance
  R : Outport
  wires:
  Resistance/1 -> R/1

== system H8_6GDL_nolineal/EMS/RL3/Subsystem ==
  Current : Inport
  Temperature : Inport  Port=2
  Resistance : Constant  Value=ems.Resistance
  R : Outport
  wires:
  Resistance/1 -> R/1

== system H8_6GDL_nolineal/HEMS1/RL/Subsystem ==
  Current : Inport
  Temperature : Inport  Port=2
  Resistance : Constant  Value=hems.Resistance
  R : Outport
  wires:
  Resistance/1 -> R/1

== system H8_6GDL_nolineal/HEMS1/RL1/Subsystem ==
  Current : Inport
  Temperature : Inport  Port=2
  Resistance : Constant  Value=hems.Resistance
  R : Outport
  wires:
  Resistance/1 -> R/1

== system H8_6GDL_nolineal/HEMS1/RL2/Subsystem ==
  Current : Inport
  Temperature : Inport  Port=2
  Resistance : Constant  Value=hems.Resistance
  R : Outport
  wires:
  Resistance/1 -> R/1

== system H8_6GDL_nolineal/HEMS1/RL3/Subsystem ==
  Current : Inport
  Temperature : Inport  Port=2
  Resistance : Constant  Value=hems.Resistance
  R : Outport
  wires:
  Resistance/1 -> R/1

== system H8_6GDL_nolineal/Modelado electromagnetico/Guidance/power_ems1 ==
  I : Inport
  Constant8 : Constant  Value=ems.Resistance
  Power : Math  Operator=magnitude^2
  Product : Product
  p(t) : Outport
  wires:
  I/1 -> Power/1
  Product/1 -> p(t)/1
  Power/1 -> Product/1
  Constant8/1 -> Product/2

== system H8_6GDL_nolineal/Modelado electromagnetico/Guidance/power_ems2 ==
  I : Inport
  Constant8 : Constant  Value=ems.Resistance
  Power : Math  Operator=magnitude^2
  Product : Product
  p(t) : Outport
  wires:
  I/1 -> Power/1
  Product/1 -> p(t)/1
  Power/1 -> Product/1
  Constant8/1 -> Product/2

== system H8_6GDL_nolineal/Modelado electromagnetico/Guidance/power_ems3 ==
  I : Inport
  Constant8 : Constant  Value=ems.Resistance
  Power : Math  Operator=magnitude^2
  Product : Product
  p(t) : Outport
  wires:
  I/1 -> Power/1
  Product/1 -> p(t)/1
  Power/1 -> Product/1
  Constant8/1 -> Product/2

== system H8_6GDL_nolineal/Modelado electromagnetico/Guidance/power_ems4 ==
  I : Inport
  Constant8 : Constant  Value=ems.Resistance
  Power : Math  Operator=magnitude^2
  Product : Product
  p(t) : Outport
  wires:
  I/1 -> Power/1
  Product/1 -> p(t)/1
  Power/1 -> Product/1
  Constant8/1 -> Product/2

== system H8_6GDL_nolineal/Modelado electromagnetico/Levitation/power_hems1 ==
  I : Inport
  Constant8 : Constant  Value=hems.Resistance
  Power : Math  Operator=magnitude^2
  Product : Product
  p(t) : Outport
  wires:
  I/1 -> Power/1
  Product/1 -> p(t)/1
  Power/1 -> Product/1
  Constant8/1 -> Product/2

== system H8_6GDL_nolineal/Modelado electromagnetico/Levitation/power_hems2 ==
  I : Inport
  Constant8 : Constant  Value=hems.Resistance
  Power : Math  Operator=magnitude^2
  Product : Product
  p(t) : Outport
  wires:
  I/1 -> Power/1
  Product/1 -> p(t)/1
  Power/1 -> Product/1
  Constant8/1 -> Product/2

== system H8_6GDL_nolineal/Modelado electromagnetico/Levitation/power_hems3 ==
  I : Inport
  Constant8 : Constant  Value=hems.Resistance
  Power : Math  Operator=magnitude^2
  Product : Product
  p(t) : Outport
  wires:
  I/1 -> Power/1
  Product/1 -> p(t)/1
  Power/1 -> Product/1
  Constant8/1 -> Product/2

== system H8_6GDL_nolineal/Modelado electromagnetico/Levitation/power_hems4 ==
  I : Inport
  Constant8 : Constant  Value=hems.Resistance
  Power : Math  Operator=magnitude^2
  Product : Product
  p(t) : Outport
  wires:
  I/1 -> Power/1
  Product/1 -> p(t)/1
  Power/1 -> Product/1
  Constant8/1 -> Product/2

== matlab function H8_6GDL_nolineal/Subsystem/Discr_Ampl1/MATLAB Function1 ==
  data: senal input; senal_discretizada output; N input; Max input; Min input
function senal_discretizada  = fcn(senal,N,Max,Min)

if(senal>Max)
    senal_discretizada=Max;
    return
elseif(senal<Min)
    senal_discretizada=Min;
    return
end

valor_escalon=(Max-Min)/(N-1);
i=Min;
 while(i<Max)
    if(i+valor_escalon/2>senal)
        senal_discretizada=i;
        return
    end
    i=i+valor_escalon;
end

      senal_discretizada=Max;
end

== matlab function H8_6GDL_nolineal/Subsystem/Discr_Ampl2/MATLAB Function1 ==
  data: senal input; senal_discretizada output; N input; Max input; Min input
function senal_discretizada  = fcn(senal,N,Max,Min)

if(senal>Max)
    senal_discretizada=Max;
    return
elseif(senal<Min)
    senal_discretizada=Min;
    return
end

valor_escalon=(Max-Min)/(N-1);
i=Min;
 while(i<Max)
    if(i+valor_escalon/2>senal)
        senal_discretizada=i;
        return
    end
    i=i+valor_escalon;
end

      senal_discretizada=Max;
end

== matlab function H8_6GDL_nolineal/Subsystem/Discr_Ampl/MATLAB Function1 ==
  data: senal input; senal_discretizada output; N input; Max input; Min input
function senal_discretizada  = fcn(senal,N,Max,Min)

if(senal>Max)
    senal_discretizada=Max;
    return
elseif(senal<Min)
    senal_discretizada=Min;
    return
end

valor_escalon=(Max-Min)/(N-1);
i=Min;
 while(i<Max)
    if(i+valor_escalon/2>senal)
        senal_discretizada=i;
        return
    end
    i=i+valor_escalon;
end

      senal_discretizada=Max;
end

== matlab function H8_6GDL_nolineal/Subsystem/Discr_Ampl3/MATLAB Function1 ==
  data: senal input; senal_discretizada output; N input; Max input; Min input
function senal_discretizada  = fcn(senal,N,Max,Min)

if(senal>Max)
    senal_discretizada=Max;
    return
elseif(senal<Min)
    senal_discretizada=Min;
    return
end

valor_escalon=(Max-Min)/(N-1);
i=Min;
 while(i<Max)
    if(i+valor_escalon/2>senal)
        senal_discretizada=i;
        return
    end
    i=i+valor_escalon;
end

      senal_discretizada=Max;
end

== matlab function H8_6GDL_nolineal/Subsystem/Discr_Ampl4/MATLAB Function1 ==
  data: senal input; senal_discretizada output; N input; Max input; Min input
function senal_discretizada  = fcn(senal,N,Max,Min)

if(senal>Max)
    senal_discretizada=Max;
    return
elseif(senal<Min)
    senal_discretizada=Min;
    return
end

valor_escalon=(Max-Min)/(N-1);
i=Min;
 while(i<Max)
    if(i+valor_escalon/2>senal)
        senal_discretizada=i;
        return
    end
    i=i+valor_escalon;
end

      senal_discretizada=Max;
end

== matlab function H8_6GDL_nolineal/Subsystem/Discr_Ampl5/MATLAB Function1 ==
  data: senal input; senal_discretizada output; N input; Max input; Min input
function senal_discretizada  = fcn(senal,N,Max,Min)

if(senal>Max)
    senal_discretizada=Max;
    return
elseif(senal<Min)
    senal_discretizada=Min;
    return
end

valor_escalon=(Max-Min)/(N-1);
i=Min;
 while(i<Max)
    if(i+valor_escalon/2>senal)
        senal_discretizada=i;
        return
    end
    i=i+valor_escalon;
end

      senal_discretizada=Max;
end

== matlab function H8_6GDL_nolineal/Subsystem/Discr_Ampl6/MATLAB Function1 ==
  data: senal input; senal_discretizada output; N input; Max input; Min input
function senal_discretizada  = fcn(senal,N,Max,Min)

if(senal>Max)
    senal_discretizada=Max;
    return
elseif(senal<Min)
    senal_discretizada=Min;
    return
end

valor_escalon=(Max-Min)/(N-1);
i=Min;
 while(i<Max)
    if(i+valor_escalon/2>senal)
        senal_discretizada=i;
        return
    end
    i=i+valor_escalon;
end

      senal_discretizada=Max;
end

== matlab function H8_6GDL_nolineal/Subsystem/Discr_Ampl7/MATLAB Function1 ==
  data: senal input; senal_discretizada output; N input; Max input; Min input
function senal_discretizada  = fcn(senal,N,Max,Min)

if(senal>Max)
    senal_discretizada=Max;
    return
elseif(senal<Min)
    senal_discretizada=Min;
    return
end

valor_escalon=(Max-Min)/(N-1);
i=Min;
 while(i<Max)
    if(i+valor_escalon/2>senal)
        senal_discretizada=i;
        return
    end
    i=i+valor_escalon;
end

      senal_discretizada=Max;
end
